simulink model "PIDkh4_controller_circle_ROS"  (R2020a)
settings: Solver=VariableStepAuto  StartTime=0.0  StopTime=15  RelTol=1e-3
undefined symbols (not defined in the file): Angular, Linear
libraries: robotlib x3, dspinverses x1, simulink x1
settings Model: Creator=FlightControlLab  LastModifiedBy=javier
settings SolverCC: SolverResetMethod=Robust
settings DataIOCC: ReturnWorkspaceOutputs=off
settings DebuggingCC: ArithmeticOperatorsInVariantConditions=warning
settings SFSimCC: SimUseLocalCustomCode=off  CustomCodeUndefinedFunction=UseInterfaceOnly
settings RTWCC: RTWUseLocalCustomCode=off

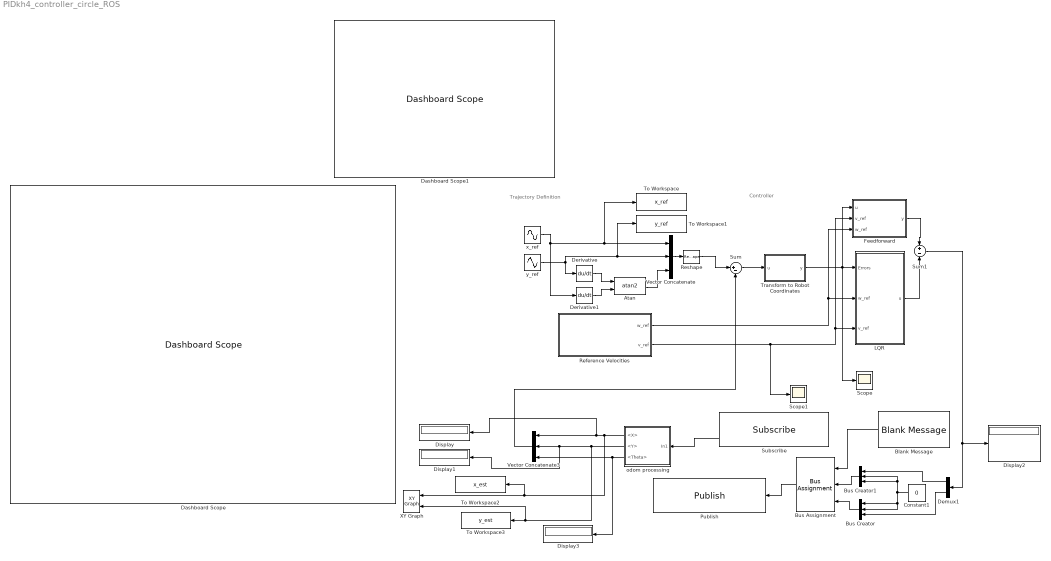
== system PIDkh4_controller_circle_ROS ==
  note: Trajectory Definition
  note: Controller
  Atan : Trigonometry  Operator=atan2
  Blank Message : robotlib/Blank Message  messageClass=Message  entityType=geometry_msgs/Twist  messageType=geometry_msgs/Twist  SampleTime=inf
  Bus Assignment : BusAssignment  AssignedSignals=Linear,Angular
  Bus Creator : BusCreator  Inputs=3
  Bus Creator1 : BusCreator  Inputs=3
  Constant1 : Constant  Value=0
  Dashboard Scope : DashboardScope
  Dashboard Scope1 : DashboardScope
  Demux1 : Demux  Outputs=2
  Derivative : Derivative
  Derivative1 : Derivative
  Display{,1..3} (4 alike) : Display
  Feedforward : MATLAB Function  TreatAsAtomicUnit=on
  LQR : Subsystem
  Publish : robotlib/Publish  topicSource=Select from ROS network  topic=/robot1/kh4_controller/cmd_vel  messageType=geometry_msgs/Twist  messageQueueLength=105
  Reference Velocities : Subsystem
  Reshape : Reshape  OutputDimensionality=Column vector (2-D)
  Scope : Scope
  Scope1 : Scope
  Subscribe : robotlib/Subscribe  topicSource=Select from ROS network  topic=/robot1/odometry/filtered  messageType=nav_msgs/Odometry  sampleTime=-1  messageQueueLength=1
  Sum : Sum  Inputs=|+-
  Sum1 : Sum  Inputs=+-
  To Workspace : ToWorkspace  VariableName=x_ref  SampleTime=-1
  To Workspace1 : ToWorkspace  VariableName=y_ref  SampleTime=-1
  To Workspace2 : ToWorkspace  VariableName=x_est  SampleTime=-1
  To Workspace3 : ToWorkspace  VariableName=y_est  SampleTime=-1
  Transform to Robot Coordinates : MATLAB Function  TreatAsAtomicUnit=on
  Vector Concatenate : Concatenate  NumInputs=3
  Vector Concatenate3 : Concatenate  NumInputs=3
  XY Graph : simulink/Sinks/XY Graph  xmin=-1  xmax=3  ymin=-1  ymax=2  st=-1
  odom processing : Subsystem
  x_ref : Sin  Amplitude=1.5  Bias=1.5  Frequency=pi/15  Phase=-pi/2  SampleTime=0
  y_ref : Sin  Amplitude=1.5  Frequency=pi/15  SampleTime=0
  wires:
  x_ref/1 -> Derivative1/1, To Workspace/1, Vector Concatenate/1
  y_ref/1 -> Derivative/1, To Workspace1/1, Vector Concatenate/2
  Transform to Robot Coordinates/1(y) -> Scope/1, Feedforward/1(u), LQR/1(Errors)
  Vector Concatenate3/1 -> Sum/2
  Vector Concatenate/1 -> Reshape/1
  Reshape/1 -> Sum/1
  Sum/1 -> Transform to Robot Coordinates/1(u)
  LQR/1(u) -> Sum1/2
  Atan/1 -> Vector Concatenate/3
  Derivative1/1 -> Atan/2
  Derivative/1 -> Atan/1
  Reference Velocities/1(w_ref) -> Feedforward/3(w_ref), LQR/2(w_ref)
  Reference Velocities/2(v_ref) -> Scope1/1, Feedforward/2(v_ref), LQR/3(v_ref)
  odom processing/1(<X>) -> Display/1, Vector Concatenate3/1, XY Graph/1, To Workspace2/1
  Bus Creator1/1 -> Bus Assignment/2
  Blank Message/1 -> Bus Assignment/1
  Bus Creator/1 -> Bus Assignment/3
  Sum1/1 -> Demux1/1, Display2/1
  Constant1/1 -> Bus Creator/2, Bus Creator/1, Bus Creator1/2, Bus Creator1/3
  Demux1/1 -> Bus Creator1/1
  Subscribe/2 -> odom processing/1(In1)
  odom processing/2(<Y>) -> XY Graph/2, To Workspace3/1, Display1/1, Vector Concatenate3/2
  Bus Assignment/1 -> Publish/1
  odom processing/3(<Theta>) -> Display3/1, Vector Concatenate3/3
  Demux1/2 -> Bus Creator/3
  Feedforward/1(y) -> Sum1/1

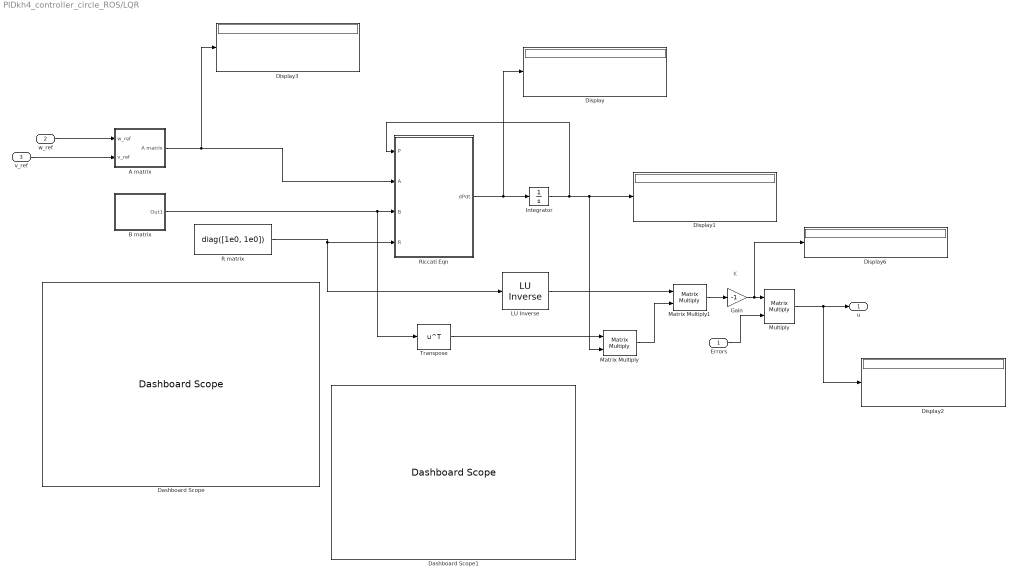
== system PIDkh4_controller_circle_ROS/LQR ==
  note: K
  Errors : Inport
  w_ref : Inport  Port=2
  v_ref : Inport  Port=3
  " LU Inverse" : dspinverses/ LU Inverse
  A matrix : Subsystem
  B matrix : Subsystem
  Dashboard Scope : DashboardScope
  Dashboard Scope1 : DashboardScope
  Display{,1..3,6} (5 alike) : Display
  Gain : Gain  Gain=-1
  Integrator : Integrator
  Matrix Multiply : Product  Multiplication=Matrix(*)
  Matrix Multiply1 : Product  Multiplication=Matrix(*)
  Multiply : Product  Multiplication=Matrix(*)
  R matrix : Constant  Value=diag([1e0, 1e0])  VectorParams1D=off
  Riccati Eqn : MATLAB Function  TreatAsAtomicUnit=on
  Transpose : Math  Operator=transpose  SignedPower=on  SaturateOnIntegerOverflow=on
  u : Outport  VectorParamsAs1DForOutWhenUnconnected=off
  wires:
  B matrix/1(Out1) -> Transpose/1, Riccati Eqn/3(B)
  R matrix/1 -> " LU Inverse"/1, Riccati Eqn/4(R)
  A matrix/1(A matrix) -> Riccati Eqn/2(A), Display3/1
  Matrix Multiply/1 -> Matrix Multiply1/2
  Transpose/1 -> Matrix Multiply/1
  w_ref/1 -> A matrix/1(w_ref)
  v_ref/1 -> A matrix/2(v_ref)
  Errors/1 -> Multiply/2
  " LU Inverse"/1 -> Matrix Multiply1/1
  Matrix Multiply1/1 -> Gain/1
  Gain/1 -> Display6/1, Multiply/1
  Riccati Eqn/1(dPdt) -> Display/1, Integrator/1
  Integrator/1 -> Riccati Eqn/1(P), Matrix Multiply/2, Display1/1
  Multiply/1 -> u/1, Display2/1

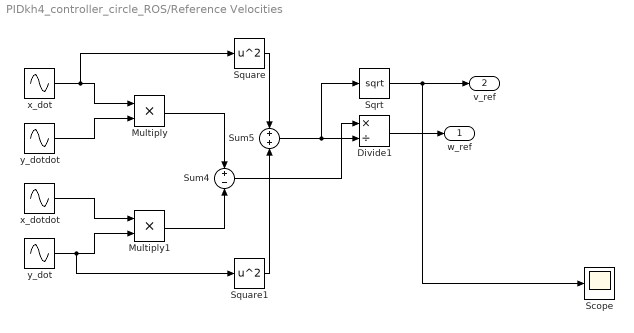
== system PIDkh4_controller_circle_ROS/Reference Velocities ==
  Divide1 : Product  Inputs=*/
  Multiply : Product
  Multiply1 : Product
  Scope : Scope
  Sqrt : Sqrt  SaturateOnIntegerOverflow=on
  Square : Math  Operator=square  SignedPower=on  SaturateOnIntegerOverflow=on
  Square1 : Math  Operator=square  SignedPower=on  SaturateOnIntegerOverflow=on
  Sum4 : Sum  Inputs=+-
  Sum5 : Sum
  x_dot : Sin  Amplitude=1.5*pi/15  Frequency=pi/15  SampleTime=0
  x_dotdot : Sin  Amplitude=-1.5*pi/15*pi/15  Frequency=pi/15  Phase=-pi/2  SampleTime=0
  y_dot : Sin  Amplitude=-1.5*pi/15  Frequency=pi/15  Phase=-pi/2  SampleTime=0
  y_dotdot : Sin  Amplitude=-1.5*pi/15*pi/15  Frequency=pi/15  SampleTime=0
  w_ref : Outport  VectorParamsAs1DForOutWhenUnconnected=off
  v_ref : Outport  Port=2  VectorParamsAs1DForOutWhenUnconnected=off
  wires:
  x_dot/1 -> Square/1, Multiply/1
  Divide1/1 -> w_ref/1
  x_dotdot/1 -> Multiply1/1
  Sum5/1 -> Divide1/2, Sqrt/1
  Square/1 -> Sum5/1
  Sum4/1 -> Divide1/1
  y_dot/1 -> Square1/1, Multiply1/2
  y_dotdot/1 -> Multiply/2
  Multiply1/1 -> Sum4/2
  Square1/1 -> Sum5/2
  Multiply/1 -> Sum4/1
  Sqrt/1 -> Scope/1, v_ref/1

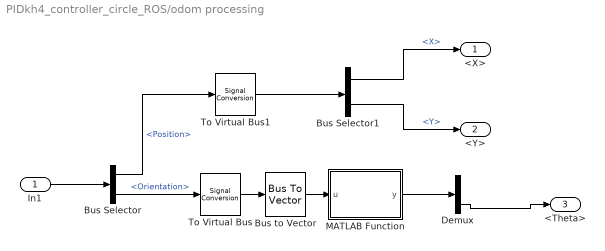
== system PIDkh4_controller_circle_ROS/odom processing ==
  In1 : Inport
  Bus Selector : BusSelector  OutputSignals=Pose.Pose.Position,Pose.Pose.Orientation
  Bus Selector1 : BusSelector  OutputSignals=X,Y
  Bus to Vector : BusToVector
  Demux : Demux  Outputs=3
  MATLAB Function : MATLAB Function  TreatAsAtomicUnit=on
  To Virtual Bus : SignalConversion  ConversionOutput=Virtual bus  OverrideOpt=off
  To Virtual Bus1 : SignalConversion  ConversionOutput=Virtual bus  OverrideOpt=off
  <X> : Outport
  <Y> : Outport  Port=2
  <Theta> : Outport  Port=3
  wires:
  In1/1 -> Bus Selector/1
  Bus Selector/1 -> To Virtual Bus1/1  "<Position>"
  To Virtual Bus/1 -> Bus to Vector/1
  Bus Selector/2 -> To Virtual Bus/1  "<Orientation>"
  To Virtual Bus1/1 -> Bus Selector1/1
  Demux/3 -> <Theta>/1
  MATLAB Function/1(y) -> Demux/1
  Bus Selector1/1 -> <X>/1  "<X>"
  Bus to Vector/1 -> MATLAB Function/1(u)
  Bus Selector1/2 -> <Y>/1  "<Y>"

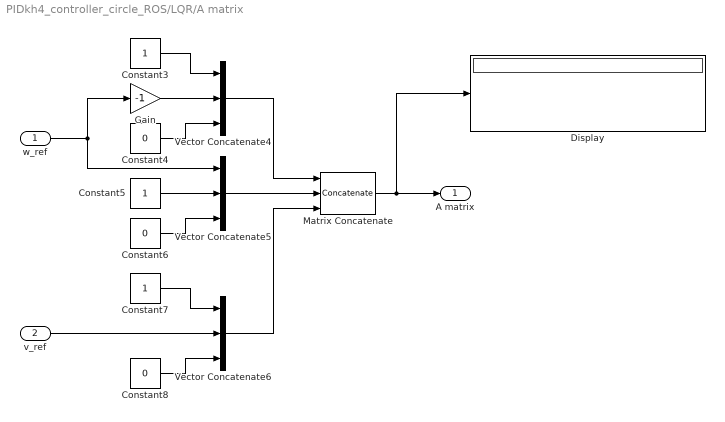
== system PIDkh4_controller_circle_ROS/LQR/A matrix ==
  w_ref : Inport
  v_ref : Inport  Port=2
  Constant3 : Constant
  Constant4 : Constant  Value=0
  Constant5 : Constant
  Constant6 : Constant  Value=0
  Constant7 : Constant
  Constant8 : Constant  Value=0
  Display : Display
  Gain : Gain  Gain=-1
  Matrix Concatenate : Concatenate  NumInputs=3  Mode=Multidimensional array  ConcatenateDimension=2
  Vector Concatenate4 : Concatenate  NumInputs=3
  Vector Concatenate5 : Concatenate  NumInputs=3
  Vector Concatenate6 : Concatenate  NumInputs=3
  A matrix : Outport  VectorParamsAs1DForOutWhenUnconnected=off
  wires:
  w_ref/1 -> Gain/1, Vector Concatenate5/1
  Gain/1 -> Vector Concatenate4/2
  Constant6/1 -> Vector Concatenate5/3
  Vector Concatenate6/1 -> Matrix Concatenate/3
  Constant4/1 -> Vector Concatenate4/3
  v_ref/1 -> Vector Concatenate6/2
  Constant7/1 -> Vector Concatenate6/1
  Vector Concatenate5/1 -> Matrix Concatenate/2
  Constant8/1 -> Vector Concatenate6/3
  Constant3/1 -> Vector Concatenate4/1
  Constant5/1 -> Vector Concatenate5/2
  Vector Concatenate4/1 -> Matrix Concatenate/1
  Matrix Concatenate/1 -> Display/1, A matrix/1

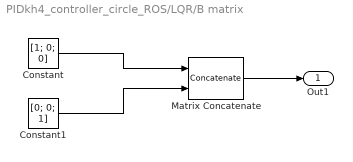
== system PIDkh4_controller_circle_ROS/LQR/B matrix ==
  Constant : Constant  Value=[1; 0; 0]  VectorParams1D=off
  Constant1 : Constant  Value=[0; 0; 1]  VectorParams1D=off
  Matrix Concatenate : Concatenate  Mode=Multidimensional array  ConcatenateDimension=2
  Out1 : Outport  VectorParamsAs1DForOutWhenUnconnected=off
  wires:
  Constant/1 -> Matrix Concatenate/1
  Matrix Concatenate/1 -> Out1/1
  Constant1/1 -> Matrix Concatenate/2

== matlab function PIDkh4_controller_circle_ROS/odom processing/MATLAB Function ==
  data: u input; y output
function y = fcn(u)

y = quat2eul(u');

== matlab function PIDkh4_controller_circle_ROS/Transform to Robot Coordinates ==
  data: u input size=[3,1]; y output size=[3,1]
function y = fcn(u)

theta = u(3);
A = [cos(theta), sin(theta), 0;
    -sin(theta), cos(theta), 0;
    0, 0, 1];

y = A*u;

== matlab function PIDkh4_controller_circle_ROS/Feedforward ==
  data: u input size=[3,1]; y output size=[2,1]; v_ref input size=1; w_ref input size=1
function y = fcn(u, v_ref, w_ref)

    e3 = u(3);
    
    y = [cos(e3)*v_ref;
        w_ref];

== matlab function PIDkh4_controller_circle_ROS/LQR/Riccati Eqn ==
  data: dPdt output size=[3,3]; P input size=[3,3]; A input size=[3,3]; B input size=[3,2]; R input size=[2,2]
function dPdt = mRiccati(P,A,B,R)


% Q = diag([0.1 0.1 0.6]);
Q = diag([5.5 5.5 216.5]);


% P2 = (A'*P - (P*B)*pinv(R)*(B'*P) + Q)*pinv(-A);

% Continuous Riccati differential equation
dPdt = A.'*P + P*A - (P*B)*inv(R)*(B.'*P) + Q;
